simulink model "system_SMA_working"  (R2018a)
settings: Solver=ode15s  StartTime=0.0  StopTime=30  MaxStep=1e-3  RelTol=1e-3
InitFcn:
  | params_SMA
values from neighbouring files (symbols this model uses):
  init = struct    [params_SMA.m]
  U = 0.5    [run.m]
undefined symbols (not defined in the file or in its folder): fluid, sma, valve
libraries: simulink x1
settings Model: Creator=Felix Welsch  LastModifiedBy=tim
settings OptimizationCC: LifeSpan=inf
settings DebuggingCC: SFExecutionAtInitializationDiag=none
settings CodeAppCC: StateflowObjectComments=on

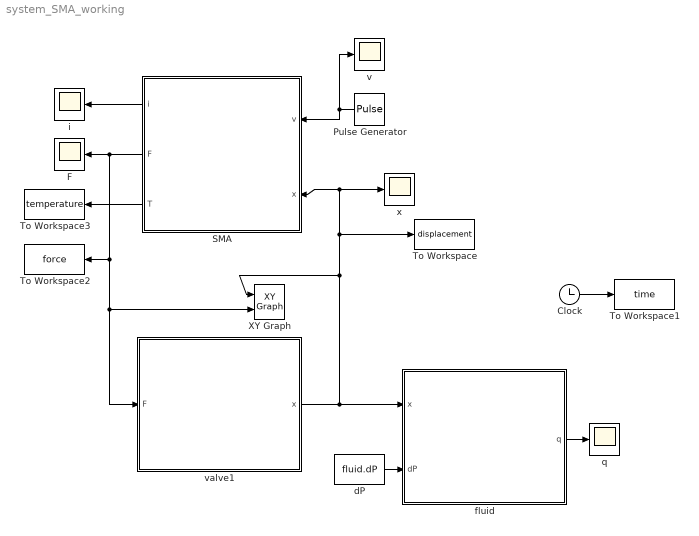
== system system_SMA_working ==
  Clock : Clock
  F : Scope
  Pulse Generator : DiscretePulseGenerator  PulseType=Time based  Amplitude=U  Period=10  PulseWidth=50  PhaseDelay=2.5
  SMA : Subsystem
  To Workspace : ToWorkspace  VariableName=displacement  SampleTime=-1
  To Workspace1 : ToWorkspace  VariableName=time  SampleTime=-1
  To Workspace2 : ToWorkspace  VariableName=force  SampleTime=-1
  To Workspace3 : ToWorkspace  VariableName=temperature  SampleTime=-1
  XY Graph : simulink/Sinks/XY Graph  xmin=0  xmax=7e-3  ymin=0  ymax=10  st=-1
  dP : Constant  Value=fluid.dP
  fluid : Subsystem
  i : Scope
  q : Scope
  "v " : Scope
  valve1 : Subsystem
  x : Scope
  wires:
  fluid/1(q) -> q/1
  dP/1 -> fluid/2(dP)
  SMA/1(i) -> i/1
  Pulse Generator/1 -> SMA/1(v), "v "/1
  SMA/2(F) -> To Workspace2/1, valve1/1(F), XY Graph/2, F/1
  Clock/1 -> To Workspace1/1
  valve1/1(x) -> fluid/1(x), To Workspace/1, x/1, SMA/2(x), XY Graph/1
  SMA/3(T) -> To Workspace3/1

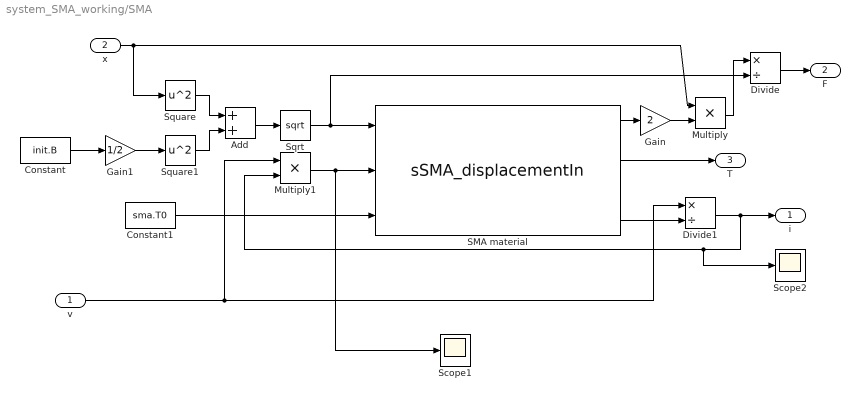
== system system_SMA_working/SMA ==
  v : Inport
  x : Inport  Port=2
  Add : Sum
  Constant : Constant  Value=init.B
  Constant1 : Constant  Value=sma.T0
  Divide : Product  Inputs=*/
  Divide1 : Product  Inputs=*/
  Gain : Gain  Gain=2
  Gain1 : Gain  Gain=1/2
  Multiply : Product
  Multiply1 : Product
  SMA material : M-S-Function  FunctionName=sSMA_displacementIn  Parameters=sma, init
      mask Display:
      | color('black');
      | patch(3*[-1 1 1 -1],1.1*[-1 -1 1 1],[1 1 1]);
      | patch([-1.6 -0.8],[-0.9 0.3],[0 0 0]);
      | patch([-0.8 1.2],[0.3 0.3],[0 0 0]);
      | patch([1.6 0.8],[0.9 -0.3],[0 0 0]);
      | patch([0.8 -1.2],[-0.3 -0.3],[0 0 0]);
      | disp('SMA');
      | 
      | color('blue');
      | port_label('input', 1, 'y [m]','texmode','on');
      | port_label('input', 2, 'J [W]','texmode','on');
      | port_label('input', 3, 'T_E [K]','texmode','on');
      | 
      | color('red');
      | port_label('output', 1, 'F [N]','texmode','on');
      | port_label('output', 2, 'x_+, x_-, x_A [-]','texmode','on');
      | port_label('output', 3, 'T [K]','texmode','on');
      | port_label('output', 4, '\epsilon [-]','texmode','on');
      | port_label('output', 5, '\sigma [Pa]','texmode','on');
      | port_label('output', 6, 'R [\Omega]','texmode','on');
  Scope1 : Scope
  Scope2 : Scope
  Sqrt : Sqrt  SaturateOnIntegerOverflow=on
  Square : Math  Operator=square  SaturateOnIntegerOverflow=on
  Square1 : Math  Operator=square  SaturateOnIntegerOverflow=on
  i : Outport
  F : Outport  Port=2
  T : Outport  Port=3
  wires:
  SMA material/1 -> Gain/1
  Multiply/1 -> Divide/1
  Gain/1 -> Multiply/2
  x/1 -> Square/1, Multiply/1
  Divide/1 -> F/1
  Square/1 -> Add/1
  Square1/1 -> Add/2
  Add/1 -> Sqrt/1
  Constant/1 -> Gain1/1
  Gain1/1 -> Square1/1
  Sqrt/1 -> Divide/2, SMA material/1
  v/1 -> Multiply1/1, Divide1/1
  Divide1/1 -> Scope2/1, Multiply1/2, i/1
  SMA material/6 -> Divide1/2
  Constant1/1 -> SMA material/3
  Multiply1/1 -> Scope1/1, SMA material/2
  SMA material/3 -> T/1

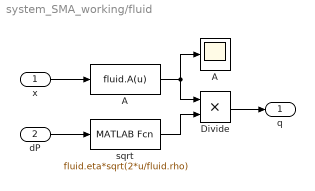
== system system_SMA_working/fluid ==
  x : Inport
  dP : Inport  Port=2
  A : MATLABFcn  MATLABFcn=fluid.A(u)
  "A " : Scope
  Divide : Product  Inputs=**
  sqrt : MATLABFcn  MATLABFcn=fluid.eta*sqrt(2*u/fluid.rho)
  q : Outport
  wires:
  x/1 -> A/1
  dP/1 -> sqrt/1
  A/1 -> "A "/1, Divide/1
  sqrt/1 -> Divide/2
  Divide/1 -> q/1

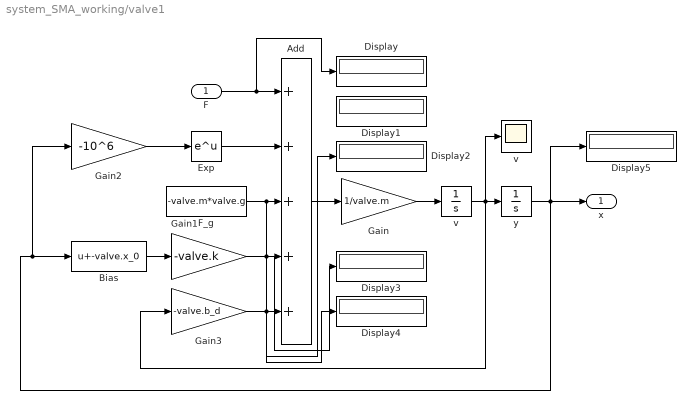
== system system_SMA_working/valve1 ==
  F : Inport
  Add : Sum  Inputs=+++++
  Bias : Bias  Bias=-valve.x_0
  Display{,1..5} (6 alike) : Display
  Exp : Math  SaturateOnIntegerOverflow=on
  F_g : Constant  Value=-valve.m*valve.g
  Gain : Gain  Gain=1/valve.m
  Gain1 : Gain  Gain=-valve.k
  Gain2 : Gain  Gain=-10^6
  Gain3 : Gain  Gain=-valve.b_d
  v : Integrator  InitialCondition=valve.v_0
  "v " : Scope
  y : Integrator  InitialCondition=valve.y_0
  x : Outport
  wires:
  F_g/1 -> Display2/1, Add/3
  y/1 -> Display5/1, x/1, Gain2/1, Bias/1
  v/1 -> "v "/1, Gain3/1, y/1
  Bias/1 -> Gain1/1
  Add/1 -> Gain/1
  Gain/1 -> v/1
  F/1 -> Display/1, Add/1
  Gain1/1 -> Display3/1, Add/4
  Gain3/1 -> Display4/1, Add/5
  Exp/1 -> Add/2
  Gain2/1 -> Exp/1
